simulink model "Commander_Stabilizer_Qdrone_wTrajTEMP"  (R2019a)
settings: Solver=ode2  StartTime=0.0  StopTime=inf  FixedStep=0.001  RelTol=1e-3  EnableMultiTasking=on
InitFcn:
  | set_param(gcs, 'ZoomFactor','FitSystem')
model workspace (MAT data in the model file):
  target_system = 1
undefined symbols (not defined in the file or in its folder): acc_calib, HIL
libraries: quarc_library x50, simulink x20, control_library x13, estimation_library x7
(part 1 of 3)
settings Model: SimulationMode=external  ExtModeTrigDuration=10000  Creator=dmadill  LastModifiedBy=user
settings SolverCC: PositivePriorityOrder=on
settings DataIOCC: LimitDataPoints=on  SaveFormat=Array  ReturnWorkspaceOutputs=off
settings OptimizationCC: LifeSpan=inf
settings DebuggingCC: SolverPrmCheckMsg=warning  SFUnexpectedBacktrackingDiag=warning  SFNoUnconditionalDefaultTransitionDiag=warning  SFExecutionAtInitializationDiag=none  ArithmeticOperatorsInVariantConditions=warning
settings HardwareCC: ProdBitPerLong=64  ProdLargestAtomicFloat=None  ProdHWDeviceType=Intel->x86-64
settings ModelReferenceCC: PropagateSignalLabelsOutOfModel=off
settings SFSimCC: SimUseLocalCustomCode=off
settings RTWCC: SystemTargetFile=quarc_linux_x64.tlc  TemplateMakefile=quarc_linux_x64_tmf  Description=QUARC Linux x64 Target  RTWUseLocalCustomCode=off
settings CodeAppCC: StateflowObjectComments=on
settings STFCustomTargetCC: TargetLibSuffix=.a  TargetPreCompLibLocation=C:\PROGRA~3\QUARC\lib\2019a\LINUX_~1\release  ConcurrentExecutionCompliant=on  SystemTargetFile=quarc_linux_x64.tlc
settings GRTTargetCC: TargetLibSuffix=.a  TargetPreCompLibLocation=C:\PROGRA~3\QUARC\lib\2019a\LINUX_~1\release  TargetLangStandard=C89/C90 (ANSI)  ParMdlRefBuildCompliant=off  CompOptLevelCompliant=off  CombineOutputUpdateFcns=off  MatFileLogging=off  CPPClassGenCompliant=off  GRTInterface=on  UseToolchainInfoCompliant=off  ExtMode=on  ExtModeMexFile=quarc_comm  ExtModeMexArgs='-w -d /tmp -uri %u -IP_address tcpip://192.168.1.157:18000', 'tcpip://192.168.1.25:17001?retries=10'
settings ConfigComp: CovMetricSettings=dw  CovHtmlReporting=on  CovSaveCumulativeToWorkspaceVar=on  CovSaveSingleToWorkspaceVar=on  CovExternalEMLEnable=off  CovSFcnEnable=off

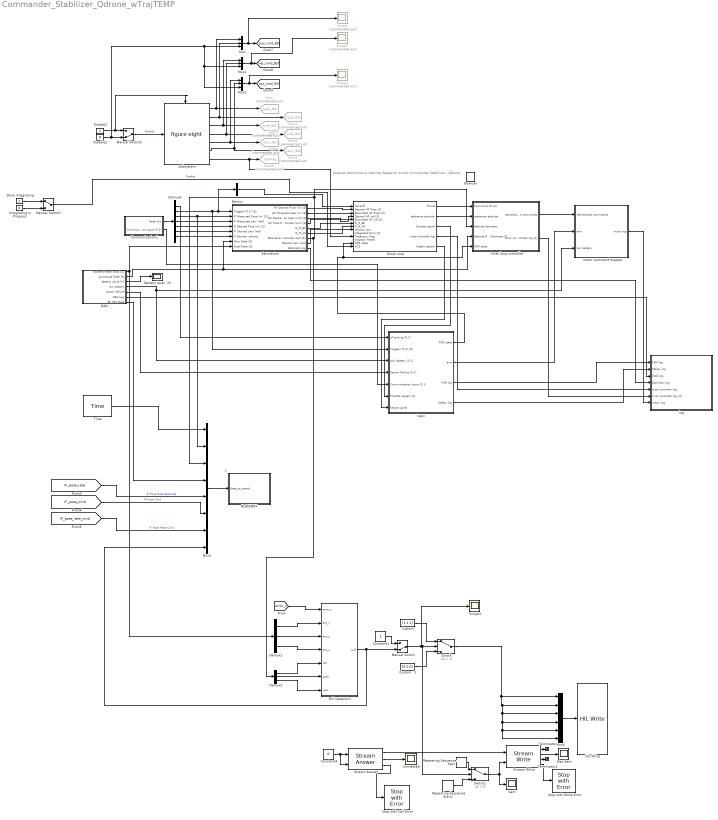
== system Commander_Stabilizer_Qdrone_wTrajTEMP ==
  note: Quanser Autonomous Vehicles Research Studio
      | Commander Stabilizer - QDrone
  note: 5
  "   Custom   " : Constant  Value=[1 1 1]
  "   Custom   1" : Constant  Value=[0 0 0]
  BLACKBOX : Subsystem
  Battery level  (V) : Scope
  Communication1 : Subsystem
  Connected : Scope
  Constant1 : Constant
  Constant4 : Constant  Value=0
  "DAQ " : Subsystem
  Demux : Demux  Outputs=3
  Demux1 : Demux  Outputs=3
  Demux2 : Demux  Outputs=3
  Demux5 : Demux  Outputs=[1 3 3 1 3 1 3]
  Disable2 : Constant  Value=0
  Done Integrating : Constant
  Enable2 : Constant
  "Estimation " : Subsystem
  Goto : Goto  Commented=on  GotoTag=xpos_8sh  TagVisibility=global
  Goto1 : Goto  Commented=on  GotoTag=ypos_8sh  TagVisibility=global
  Goto2 : Goto  Commented=on  GotoTag=xvel_8sh  TagVisibility=global
  Goto3 : Goto  Commented=on  GotoTag=yvel_8sh  TagVisibility=global
  Goto4 : Goto  Commented=on  GotoTag=xacc_8sh  TagVisibility=global
  Goto5 : Goto  Commented=on  GotoTag=yacc_8sh  TagVisibility=global
  Goto6 : Goto  Commented=on  GotoTag=trajFlag  TagVisibility=global
  HIL Write : quarc_library/Data Acquisition/Generic/Immediate I//O/HIL Write  object_name=HIL-1  analog_channels=[]  pwm_channels=[]  digital_channels=[5:7 9:23]  other_channels=[]  sample_time=-1  active=off  vector_input=on
      settings: SourceProductName=The database C:\Users\user\AppData\Roaming\MathWorks\MATLAB\R2017a\slblocks_master.db is locked, or a table in the database is locked. (database is locked)
  "Inner loop controller " : Subsystem
  Integrating in Progress : Constant  Value=0
  Manual Switch : ManualSwitch  CurrentSetting=0
  Manual Switch1 : ManualSwitch
  Manual Switch3 : ManualSwitch  CurrentSetting=0
  Mux : Mux  Inputs=3
  Mux1 : Mux  Inputs=3
  Mux2 : Mux  Inputs=3
  Mux3 : Mux  Inputs=[1 3 3 6 3 3 3 1]
  Mux4 : Mux  Inputs=6
  Outer loop : Subsystem
  Pull Detector1 : Subsystem
  Quanser : quarc_library/Logos/Quanser
  Repeating Sequence Stair : simulink/Sources/Repeating Sequence Stair  OutValues=[255 255 1 7 3 30 0 0 0 0 214].'  tsamp=-1  OutMin=[0]  OutMax=[]  OutDataTypeStr=fixdt(0,8,0)  OutputDataTypeScalingMode=Specify via dialog  OutDataType=fixdt(0,8,0)  ConRadixGroup=Best Precision: Vector-wise  OutScaling=[]
  Repeating Sequence Stair1 : simulink/Sources/Repeating Sequence Stair  OutValues=[255 255 1 7 3 30 255 3 0 0 212].'  tsamp=-1  OutMin=[0]  OutMax=[]  OutDataTypeStr=fixdt(0,8,0)  OutputDataTypeScalingMode=Specify via dialog  OutDataType=fixdt(0,8,0)  ConRadixGroup=Best Precision: Vector-wise  OutScaling=[]
  Scope : Scope  Commented=on
  Scope1 : Scope  Commented=on
  Scope2 : Scope  Commented=on
  Scope3 : Scope
  Sent : Scope
  Stop with Call Error : quarc_library/Sinks/Error Handling/Stop with Error  message_type=Interpret input as error code  message=Error occurred
      settings: SourceProductName=QUARC Targets
  Stop with Write Error : quarc_library/Sinks/Error Handling/Stop with Error  message_type=Interpret input as error code  message=Error occurred
      settings: SourceProductName=QUARC Targets
  Stream Answer : quarc_library/Communications/Intermediate/Stream Answer  uri_source=Specify via dialog (do not evaluate)  uri=serial://localhost:1?sndsize='16',baud='9600',word='8'  apply_uri_to_all_configs=on  send_buffer_size=128  receive_buffer_size=128  byte_order=little endian (Intel - LSB first)  sample_time=qc_get_step_size  active=off
      settings: AttributesFormatString="\"serial://localhost:1?sndsize='16',baud='9600',word='8'\""  SourceProductName=QUARC Targets
  Stream Write : quarc_library/Communications/Intermediate/Stream Write  optimization=Minimizing latency  send_dims=off
      settings: SourceProductName=QUARC Targets
  Subsystem : control_library/figure eight  TrajTime=8
  Switch : Switch  Criteria=u2 > Threshold
  Switch1 : Switch  Criteria=u2 > Threshold
  Terminator : Terminator
  Terminator1 : Terminator
  Time : quarc_library/Sources/Time/Time  time_source=Wall clock  sample_time=qc_get_step_size
  Was Sent : Scope
  "log " : Subsystem
  logic : Subsystem
  motor command mapper : Subsystem
  tag scope: acc_cmd_8sh=global, pos_cmd_8sh=global, vel_cmd_8sh=global
  wires:
  Demux5/3 -> "Estimation "/2(IF Measured Pose (m) [3]), Mux3/2
  Communication1/1(Data Out) -> Demux5/1
  Demux5/2 -> logic/2(Triggers (0,1) [3]), Demux/1, "Estimation "/1(Triggers (0,1) [3])
  "DAQ "/1(accelerometer Data [3]) -> "Estimation "/8(Accel Data [3]), Demux1/1
  Demux5/5 -> "Estimation "/4(IF Desired Pose (m) [3])
  Demux5/7 -> "Estimation "/6(IF Desired velocity)
  Demux5/4 -> "Estimation "/3(IF Measured yaw (rad))
  Demux5/6 -> "Estimation "/5(IF Desired yaw (rad))
  "DAQ "/2("gyroscope Data [3] ") -> "Estimation "/7(Gyro Data [3]), "Inner loop controller "/4(Attitude Rate Estimate [3])
  "Estimation "/1(HF Desired Pose (m) [3]) -> Outer loop/2(Desired HF Pose [3])
  "Estimation "/2(HF Pose Estimate (m) [3]) -> Outer loop/3(Estimated HF Pose [3])
  "Estimation "/3(HF Desired Pose rate (m/s) [3]) -> Outer loop/4(Desired HF vel [3])
  "Estimation "/4(HF Pose Rate Estimate (m/s) [3]) -> Outer loop/5(Estimated HF vel [3])
  "Estimation "/6(IF_R_HF) -> Outer loop/7(IF_R_HF)
  Demux5/1 -> logic/1(isTracking (0,1))
  logic/1("FSM state ") -> Outer loop/12("FSM state "), "Inner loop controller "/5(FSM state)
  "DAQ "/5(sensor failure) -> logic/4(Sensor Failure (0,1))
  "DAQ "/4(low battery) -> logic/3(Low Battery (0,1)), motor command mapper/3(low battery)
  Outer loop/1(Thrust) -> "Inner loop controller "/1(Command thrust)
  Communication1/2(Communication Issue (0,1)) -> logic/5(Communication Issue (0,1))
  "Inner loop controller "/1(Generalized commands) -> motor command mapper/1(Generalized commands)
  logic/2(arm) -> motor command mapper/2(arm)
  Outer loop/2(reference attitude) -> "Inner loop controller "/2(reference attitude)
  "Estimation "/7(Attitude Estimate (rad) [3]) -> Demux2/1, Mux3/3, "Inner loop controller "/3(Attitude Estimate)
  "DAQ "/6(DAQ Log) -> "log "/3(DAQ Log)
  "Estimation "/9(Estimator log) -> "log "/4(Estimator log)
  motor command mapper/1(motor log) -> "log "/7(motor log)
  Outer loop/4("outer controler log ") -> "log "/5("outer controler log ")
  "Inner loop controller "/2(inner controller log [4]) -> "log "/6(inner controller log [4])
  logic/3("FSM log ") -> "log "/1(FSM log)
  logic/4(Safety log) -> "log "/2(Safety log)
  "DAQ "/3(Battery Level (V)) -> Battery level  (V)/1
  Outer loop/5(height signals) -> logic/7(height signal)
  "Estimation "/5(IF_R_BF) -> Outer loop/6(IF_R_BF)
  "Estimation "/8(Desired Yaw (rad)) -> Outer loop/8(desired yaw)
  Outer loop/3(throttle signal) -> logic/6(Throttle signals [3])
  Manual Switch3/1 -> Subsystem/1  "Enable"
  Subsystem/5 -> Mux2/1, Goto4/1
  Mux/1 -> Scope/1, [pos_cmd_8sh]
  Mux1/1 -> Scope1/1, [vel_cmd_8sh]
  Subsystem/7 -> Outer loop/10(Trajectory Flag), Goto6/1
  Subsystem/6 -> Goto5/1, Mux2/2
  Subsystem/3 -> Mux1/1, Goto2/1
  Mux2/1 -> Scope2/1, [acc_cmd_8sh]
  Subsystem/4 -> Mux1/2, Goto3/1
  Disable2/1 -> Manual Switch3/2, Mux2/3, Mux1/3, Mux/3
  Subsystem/1 -> Mux/1, Goto/1
  Subsystem/2 -> Mux/2, Goto1/1
  Enable2/1 -> Manual Switch3/1, Subsystem/Enable
  Mux3/1 -> BLACKBOX/1("data_to_rocard ")
  Time/1 -> Mux3/1
  "DAQ "/7(BF IMU Data) -> Mux3/4
  [IF_pose_rate] -> Mux3/5  "IF Pose Rate Estimate"
  [IF_pose_cmd] -> Mux3/6  "IF Pose Cmd"
  [IF_pose_rate_cmd] -> Mux3/7  "IF Pose Rate Cmd"
  Demux/2 -> Outer loop/1(Takeoff)
  Done Integrating/1 -> Manual Switch1/1
  Integrating in Progress/1 -> Manual Switch1/2
  Manual Switch1/1 -> Outer loop/13(In13)  "Enable"
  Stream Write/1 -> Terminator/1
  Stream Answer/1 -> Stream Write/1
  Pull Detector1/1(pull) -> Mux3/8, Manual Switch/2
  Stream Write/2 -> Was Sent/1
  Repeating Sequence Stair1/1 -> Switch1/3
  Switch1/1 -> Stream Write/2, Sent/1
  Stream Answer/2 -> Connected/1
  Stream Write/4 -> Stop with Write Error/1
  Repeating Sequence Stair/1 -> Switch1/1
  Constant4/1 -> Stream Answer/1, Stream Answer/2
  Stream Answer/3 -> Stop with Call Error/1
  Constant1/1 -> Manual Switch/1
  Manual Switch/1 -> Switch1/2, Switch/2, Scope3/1
  "   Custom   1"/1 -> Switch/3
  Mux4/1 -> HIL Write/1
  "   Custom   "/1 -> Switch/1
  Switch/1 -> Mux4/6, Mux4/5, Mux4/4, Mux4/3, Mux4/2, Mux4/1
  Stream Write/3 -> Terminator1/1
  [error_z] -> Pull Detector1/1(error_z)
  Demux1/1 -> Pull Detector1/2(acc_x)
  Demux1/2 -> Pull Detector1/3(acc_y)
  Demux1/3 -> Pull Detector1/4(acc_z)
  Demux2/1 -> Pull Detector1/5(roll)
  Demux2/2 -> Pull Detector1/6(pitch)
  Demux2/3 -> Pull Detector1/7(yaw)

== system Commander_Stabilizer_Qdrone_wTrajTEMP/BLACKBOX ==
  "data_to_rocard " : Inport
  To Host File : quarc_library/Sinks/To Host/To Host File  file_name=saved_data/%m/record_data_%{date}_%{time}.mat  variable_name=optitack_imu_data  decimation=1  sample_time=-1  file_format=MAT-file v.5  options=No header or footer  append=off  final_file_name=saved_data/Commander_Stabilizer_Qdrone_wTrajTEMP/record_data_30-Mar-2021_18-24-55.mat  bitrate=2000000
  wires:
  "data_to_rocard "/1 -> To Host File/1

== system Commander_Stabilizer_Qdrone_wTrajTEMP/Communication1 ==
  note: Argument (- IP_address ) is set at the MEX-file arguments found at Model Configuration Properties > Code Generation > Interface
      |
      | Format:
      | tcpip://192.168.2.H:18000
      | where H is the last digits of your ground station's IP address (use ipconfig in a command prompt to find it out).
  Constant : Constant
  Detect Communication Loss : Subsystem
  Memory : Memory  InheritSampleTime=on  LinearizeMemory=on  LinearizeAsDelay=on
  Model Argument : quarc_library/Sources/Signals/Model Argument  argument_name=IP_address  has_value=on  data_type_mode=Specify via dialog  data_type=char  max_length=80  variable_size=off
      settings: AttributesFormatString=(-%<argument_name>)  SourceProductName=QUARC Targets
  Select Timestamp received and send back immediately (for calculating loopback time) : Selector  InputPortWidth=16  IndexOptions=Index vector (dialog)  Indices=[16]  OutputSizes=1
  Select the rest of the data : Selector  InputPortWidth=16  IndexOptions=Index vector (dialog)  Indices=[1:15]  OutputSizes=1
  Stream Client : quarc_library/Communications/Basic/Stream Client  uri_source=External input port  uri=tcpip://192.168.2.3:18669  apply_uri_to_all_configs=on  send_buffer_size=128  receive_buffer_size=128  byte_order=little endian (Intel - LSB first)  optimization=Minimum latency  send_options=Send most recent data  receive_options=Receive most recent data  default_value=zeros(1,16)  sample_time=qc_get_step_size  active=off  implementation=Use blocking I/O in a separate thread  send_fifo_size=128  receive_fifo_size=128  send_priority=0  receive_priority=0  send_dimensions=off  receive_dimensions=off  max_dimensions=-1  data_type=Inherited via back propagation  type_expr=BusObject
  String Display : quarc_library/Strings/String Display  alignment=center  display_mode=Single line  sample_time=-1
      settings: SourceProductName=QUARC Targets
  Terminator1 : Terminator
  Terminator2 : Terminator
  Data Out : Outport
  Communication Issue (0,1) : Outport  Port=2
  wires:
  Stream Client/5 -> Terminator2/1
  Model Argument/1 -> Stream Client/3, String Display/1
  Constant/1 -> Stream Client/2
  Stream Client/3 -> Terminator1/1
  Stream Client/4 -> Detect Communication Loss/3(Data Out), Select Timestamp received and send back immediately (for calculating loopback time)/1, Select the rest of the data/1
  Memory/1 -> Stream Client/1
  Stream Client/1 -> Detect Communication Loss/1(State)
  Stream Client/2 -> Detect Communication Loss/2(Error)
  Detect Communication Loss/1(Communication Issue) -> Communication Issue (0,1)/1
  Select the rest of the data/1 -> Data Out/1
  Select Timestamp received and send back immediately (for calculating loopback time)/1 -> Memory/1

== system Commander_Stabilizer_Qdrone_wTrajTEMP/DAQ  ==
  note: Read the sensors and battery voltage
  note: Gyro and Accel data rate at 1000Hz
  Accel (m/s/s) [3] : Selector  InputPortWidth=6  IndexOptions=Index vector (dialog)  Indices=[4:6]  OutputSizes=1
  "Battery Level, Accelrometer and Gyroscope" : quarc_library/Data Acquisition/Generic/Immediate I//O/HIL Read  Priority=1  object_name=HIL-1  analog_channels=[4]  encoder_channels=[]  digital_channels=[]  other_channels=[3000:3002 4000:4002]  sample_time=qc_get_step_size  active=on  vector_output=on  data_type_mode=Inherit via back propagation  encoder_data_type=double  digital_data_type=boolean
      settings: SourceProductName=The database C:\Users\user\AppData\Roaming\MathWorks\MATLAB\R2017a\slblocks_master.db is locked, or a table in the database is locked. (database is locked)
  Check Battery level : Subsystem
  Conversion : Gain  Gain=11.2
  Gyro (rad/s) [3] : Selector  InputPortWidth=6  IndexOptions=Index vector (dialog)  Indices=[1:3]  OutputSizes=1
  HIL Initialize : quarc_library/Data Acquisition/Generic/Configuration/HIL Initialize  object_name=HIL-1  board_type=qdrone  board_number=0  board_options=gyro_fs=2000;gyro_rate=1000;gyro_os=4;accel_fs=16;accel_rate=400;accel_os=4;baro_os=4096  exclusive=off  active=on  hardware_clocks=[]  clock_modes=[]  initial_clock_frequencies=[]  set_clock_params_at_start=off  set_clock_params_at_switch_in=off  set_clock_frequencies_at_start=off  set_clock_frequencies_at_switch_in=off  analog_input_channels=[0:4]  analog_input_configurations=[]  analog_input_maximums=[3.3]  analog_input_minimums=[0]  set_analog_input_params_at_start=off  set_analog_input_params_at_switch_in=off  analog_output_channels=[]  analog_output_maximums=[]  analog_output_minimums=[]  initial_analog_outputs=[]  final_analog_outputs=[]  watchdog_analog_outputs=[]  set_analog_output_params_at_start=off  set_analog_output_params_at_switch_in=off  set_analog_outputs_at_start=off  set_analog_outputs_at_switch_in=off  set_analog_outputs_at_terminate=off  set_analog_outputs_at_switch_out=off  set_analog_outputs_on_watchdog=off  digital_input_channels=[]  digital_output_channels=[5:7 9:23]  digital_output_configuration=[]  initial_digital_outputs=[0]  final_digital_outputs=[0]  watchdog_digital_outputs=[]  set_digital_output_params_at_start=off  set_digital_output_params_at_switch_in=off  set_digital_outputs_at_start=on  set_digital_outputs_at_switch_in=off  set_digital_outputs_at_terminate=on  set_digital_outputs_at_switch_out=off  set_digital_outputs_on_watchdog=off  encoder_channels=[0:2]  quadrature=[4]  encoder_filter_frequency=50e6/1  initial_encoder_counts=[0]  set_encoder_params_at_start=on  set_encoder_params_at_switch_in=off  set_encoder_counts_at_start=on  set_encoder_counts_at_switch_in=off  pwm_channels=[0:3]  pwm_modes=[4]  pwm_frequency=2000  pwm_configuration=[0]  pwm_alignment=[0]  pwm_polarity=[1]  pwm_leading_deadband=[]  pwm_trailing_deadband=[]  initial_pwm_outputs=[0]  final_pwm_outputs=[0]  watchdog_pwm_outputs=[0]  set_pwm_params_at_start=on  set_pwm_params_at_switch_in=off  set_pwm_outputs_at_start=on  set_pwm_outputs_at_switch_in=off  set_pwm_outputs_at_terminate=on  set_pwm_outputs_at_switch_out=off  set_pwm_outputs_on_watchdog=off  other_output_channels=[]  initial_other_outputs=[]  final_other_outputs=[]  watchdog_other_outputs=[]  set_other_outputs_at_start=off  set_other_outputs_at_switch_in=off  set_other_outputs_at_terminate=off  set_other_outputs_at_switch_out=off  set_other_outputs_on_watchdog=off
      settings: SourceProductName=The database C:\Users\user\AppData\Roaming\MathWorks\MATLAB\R2017a\slblocks_master.db is locked, or a table in the database is locked. (database is locked)
  Mux : Mux  Inputs=5
  Sensor Failure Monitoring : Subsystem
  accelerometer Data [3] : Outport
  "gyroscope Data [3] " : Outport  Port=2
  Battery Level (V) : Outport  Port=3
  low battery : Outport  Port=4
  sensor failure : Outport  Port=5
  DAQ Log : Outport  Port=6
  BF IMU Data : Outport  Port=7
  wires:
  Mux/1 -> DAQ Log/1
  Sensor Failure Monitoring/1(Sensor Failure) -> sensor failure/1, Mux/1
  Accel (m/s/s) [3]/1 -> accelerometer Data [3]/1, Sensor Failure Monitoring/2(Accel Data [3]1), Mux/5
  "Battery Level, Accelrometer and Gyroscope"/2 -> BF IMU Data/1, Accel (m/s/s) [3]/1, Gyro (rad/s) [3]/1
  Check Battery level/1(Low Battery) -> low battery/1, Mux/3
  "Battery Level, Accelrometer and Gyroscope"/1 -> Conversion/1
  Conversion/1 -> Mux/2, Battery Level (V)/1, Check Battery level/1(Battery level)
  Gyro (rad/s) [3]/1 -> "gyroscope Data [3] "/1, Sensor Failure Monitoring/1(Gyro Data [3]), Mux/4

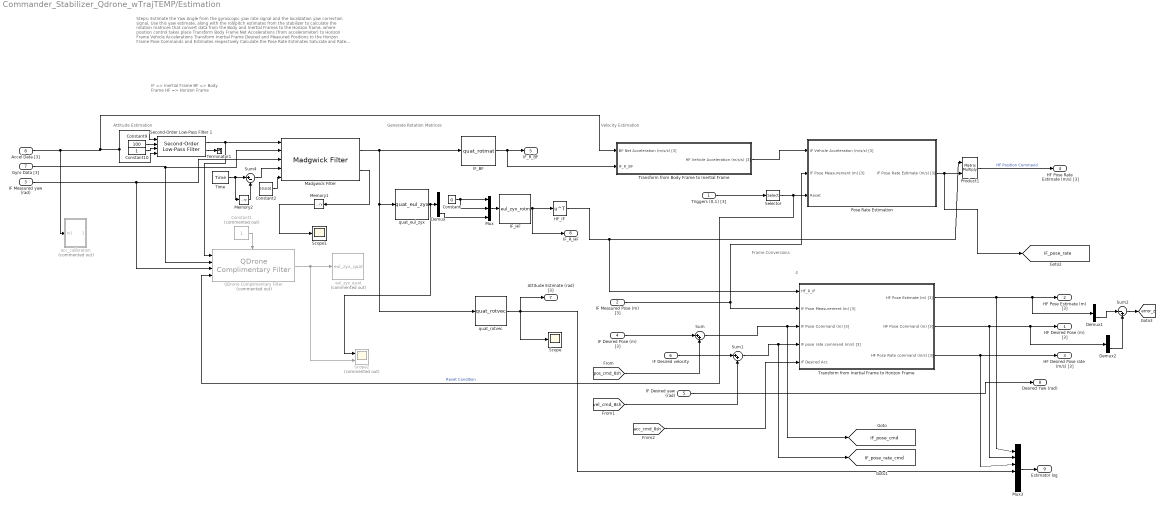
== system Commander_Stabilizer_Qdrone_wTrajTEMP/Estimation  ==
  note: IF => Inertial Frame
      | BF => Body Frame
      | HF => Horizon Frame
  note: 4
  note: Steps:
      |
      | Estimate the Yaw Angle from the gyroscopic yaw rate signal and the localization yaw correction signal.
      | Use this yaw estimate, along with the roll/pitch estimates from the stabilizer to calculate the rotation matrices that convert data from the Body and Inertial Frames to the Horizon frame, where position control takes place
      | Transform Body Frame Net Accelerations (from accelerometer) to Horizon Frame Vehicle Accelerations
      | Transform Inertial Frame Desired and Measured Positions to the Horizon Frame Pose Commands and Estimates respectively
      | Calculate the Pose Rate Estimates
      | Saturate and Rate Limit the IF Desired Pose based on workspace limitations
  note: Attitude Estimation
  note: Generate Rotation Matrices
  note: Velocity Estimation
  note: Frame Conversions
  Triggers (0,1) [3] : Inport
  IF Measured Pose (m) [3] : Inport  Port=2
  IF Measured yaw (rad) : Inport  Port=3
  IF Desired Pose (m) [3] : Inport  Port=4
  IF Desired yaw (rad) : Inport  Port=5
  IF Desired velocity : Inport  Port=6
  Gyro Data [3] : Inport  Port=7
  Accel Data [3] : Inport  Port=8
  Constant : Constant  Value=0
  Constant1 : Constant  Commented=on
  Constant10 : Constant
  Constant2 : Constant  Value=[0;0;0]
  Constant9 : Constant  Value=100
  Demux : Demux  Outputs=3
  Demux1 : Demux  Outputs=3
  Demux2 : Demux  Outputs=3
  HF_IF : Math  Operator=transpose  SaturateOnIntegerOverflow=on
  IF_BF : estimation_library/quat_rotmat
  IF_HF : estimation_library/eul_zyx_rotm
  Madgwick Filter : estimation_library/Madgwick Filter  beta=0.0453*0.1  zeta=0  acc_tol=1.1*9.78909*1e3
  Memory1 : Memory  InitialCondition=[0, 0, 0]  InheritSampleTime=on
  Memory2 : Memory  InheritSampleTime=on
  Mux : Mux  Inputs=3
  Mux3 : Mux  Inputs=6
  Pose Rate Estimation : Subsystem
  Product1 : Product  Multiplication=Matrix(*)
  QDrone Complimentary Filter : estimation_library/QDrone Complimentary Filter  Commented=on  SystemSampleTime=-1
  Scope : Scope
  Scope1 : Scope
  Scope2 : Scope  Commented=on  NumInputPorts=2
  Second-Order Low-Pass Filter 1 : quarc_library/Continuous/Second-Order Low-Pass Filter  params_source=External (input ports)  input_width=50  input_zeta=1  input_init=0
      settings: SourceProductName=The database C:\Users\user\AppData\Roaming\MathWorks\MATLAB\R2017a\slblocks_master.db is locked, or a table in the database is locked. (database is locked)
  Selector : Selector  InputPortWidth=3  IndexOptions=Index vector (dialog)  Indices=[2]  OutputSizes=1
  Sum : Sum  Inputs=|++
  Sum1 : Sum  Inputs=|++
  Sum2 : Sum  Inputs=|-+
  Sum4 : Sum  Inputs=|+-
  Terminator1 : Terminator
  Time : quarc_library/Sources/Time/Time  time_source=Wall clock  sample_time=qc_get_step_size
  Transform from Body Frame to Inertial Frame : Subsystem
  Transform from Inertial Frame to Horizon Frame : Subsystem
  acc_calibration : Subsystem  Commented=on
  eul_zyx_quat : estimation_library/eul_zyx_quat  Commented=on
  quat_eul_zyx : estimation_library/quat_eul_zyx
  quat_rotvec : estimation_library/quat_rotvec
  HF Desired Pose (m) [3] : Outport
  HF Pose Estimate (m) [3] : Outport  Port=2
  HF Desired Pose rate (m/s) [3] : Outport  Port=3
  HF Pose Rate Estimate (m/s) [3] : Outport  Port=4
  IF_R_BF : Outport  Port=5
  IF_R_HF : Outport  Port=6
  Attitude Estimate (rad) [3] : Outport  Port=7
  Desired Yaw (rad) : Outport  Port=8
  Estimator log : Outport  Port=9
  tag scope: IF_pose_cmd=global, IF_pose_rate=global, IF_pose_rate_cmd=global, error_z=global
  wires:
  IF Measured Pose (m) [3]/1 -> Transform from Inertial Frame to Horizon Frame/2(IF Pose Measurement (m) [3]), Pose Rate Estimation/2(IF Pose Measurement (m) [3])
  Triggers (0,1) [3]/1 -> Selector/1
  Transform from Inertial Frame to Horizon Frame/2(HF Pose Command (m) [3]) -> Mux3/2, Demux2/1, HF Desired Pose (m) [3]/1
  Transform from Body Frame to Inertial Frame/1(HF Vehicle Acceleration (m/s/s) [3]) -> Pose Rate Estimation/1(IF Vehicle Acceleration (m/s/s) [3])
  Selector/1 -> QDrone Complimentary Filter/4, Pose Rate Estimation/3(Reset)  "Reset Condition"
  IF Desired Pose (m) [3]/1 -> Sum/1
  IF Desired velocity/1 -> Sum1/1
  Transform from Inertial Frame to Horizon Frame/3(HF Pose Rate command (m/s) [3]) -> HF Desired Pose rate (m/s) [3]/1, Mux3/3
  Memory2/1 -> Sum4/2
  Time/1 -> Memory2/1, Sum4/1
  Sum4/1 -> Madgwick Filter/4
  Madgwick Filter/2 -> Memory1/1
  Gyro Data [3]/1 -> Madgwick Filter/2, QDrone Complimentary Filter/2
  quat_eul_zyx/1 -> Scope2/1, Demux/1
  Constant/1 -> Mux/2, Mux/1
  Mux/1 -> IF_HF/1
  IF_HF/1 -> IF_R_HF/1, HF_IF/1
  HF_IF/1 -> Product1/1, Transform from Inertial Frame to Horizon Frame/1(HF_R_IF)
  Constant10/1 -> Second-Order Low-Pass Filter 1/3
  Constant9/1 -> Second-Order Low-Pass Filter 1/2
  Second-Order Low-Pass Filter 1/1 -> Madgwick Filter/1, QDrone Complimentary Filter/1
  Second-Order Low-Pass Filter 1/2 -> Terminator1/1
  Mux3/1 -> Estimator log/1
  Transform from Inertial Frame to Horizon Frame/1(HF Pose Estimate (m) [3]) -> Demux1/1, HF Pose Estimate (m) [3]/1, Mux3/1
  quat_rotvec/1 -> Attitude Estimate (rad) [3]/1, Scope/1, Mux3/4
  Memory1/1 -> Scope1/1
  IF Desired yaw (rad)/1 -> Desired Yaw (rad)/1
  IF Measured yaw (rad)/1 -> Madgwick Filter/3, QDrone Complimentary Filter/3
  Constant1/1 -> QDrone Complimentary Filter/Enable
  QDrone Complimentary Filter/1 -> Scope2/2, eul_zyx_quat/1
  Product1/1 -> HF Pose Rate Estimate (m/s) [3]/1  "HF Position Command"
  IF_BF/1 -> Transform from Body Frame to Inertial Frame/2(IF_R_BF), IF_R_BF/1
  Demux/3 -> Mux/3
  Pose Rate Estimation/1(IF Pose Rate Estimate (m/s) [3]) -> [IF_pose_rate], Product1/2
  Sum/1 -> [IF_pose_cmd], Transform from Inertial Frame to Horizon Frame/3(IF Pose Command (m) [3])
  [pos_cmd_8sh] -> Sum/2
  Sum1/1 -> [IF_pose_rate_cmd], Transform from Inertial Frame to Horizon Frame/4(IF pose rate command (m/s) [3])
  [vel_cmd_8sh] -> Sum1/2
  [acc_cmd_8sh] -> Transform from Inertial Frame to Horizon Frame/5(IF Desired Acc)
  Constant2/1 -> Madgwick Filter/5
  Accel Data [3]/1 -> acc_calibration/1(In1), Second-Order Low-Pass Filter 1/1, Second-Order Low-Pass Filter 1/4, Transform from Body Frame to Inertial Frame/1(BF Net Acceleration (m/s/s) [3])
  Sum2/1 -> [error_z]
  Demux2/3 -> Sum2/2
  Demux1/3 -> Sum2/1
  Madgwick Filter/1 -> quat_rotvec/1, quat_eul_zyx/1, IF_BF/1

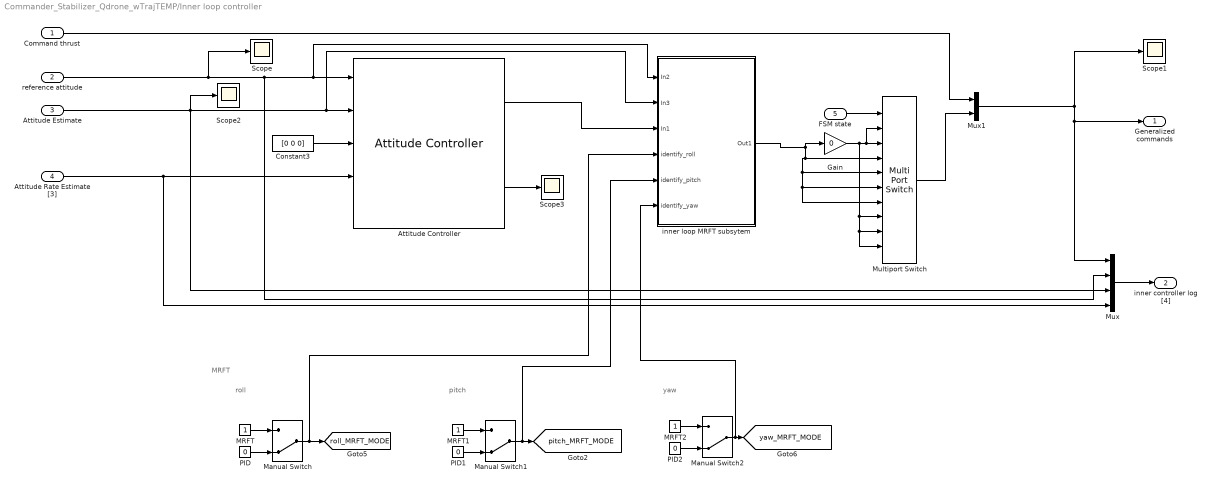
== system Commander_Stabilizer_Qdrone_wTrajTEMP/Inner loop controller  ==
  note: MRFT
  note: pitch
  note: roll
  note: yaw
  Command thrust : Inport
  reference attitude : Inport  Port=2
  Attitude Estimate : Inport  Port=3
  Attitude Rate Estimate [3] : Inport  Port=4
  FSM state : Inport  Port=5
  Attitude Controller : control_library/Attitude Controller  P_x=1.3852  I_x=0  D_x=0.1564  P_y=1.3542  I_y=0  D_y=0.1529  P_z=0.6  I_z=0  D_z=0.12  velRef=off  LowPassPID=off  T_lowpass=0
  Constant3 : Constant  Value=[0 0 0]
  Gain : Gain  Gain=0
  MRFT : Constant
  MRFT1 : Constant
  MRFT2 : Constant
  Manual Switch : ManualSwitch  CurrentSetting=0
  Manual Switch1 : ManualSwitch  CurrentSetting=0
  Manual Switch2 : ManualSwitch  CurrentSetting=0
  Multiport Switch : MultiPortSwitch  Inputs=9
  Mux : Mux
  Mux1 : Mux  Inputs=2
  PID : Constant  Value=0
  PID1 : Constant  Value=0
  PID2 : Constant  Value=0
  Scope{,1..3} (4 alike) : Scope
  inner loop MRFT subsytem : Subsystem
  Generalized commands : Outport
  inner controller log [4] : Outport  Port=2
  tag scope: pitch_MRFT_MODE=global, roll_MRFT_MODE=global, yaw_MRFT_MODE=global
  wires:
  Constant3/1 -> Attitude Controller/3
  reference attitude/1 -> Scope/1, Mux/2, inner loop MRFT subsytem/1(In2), Attitude Controller/1
  Command thrust/1 -> Mux1/1
  Mux/1 -> inner controller log [4]/1
  Attitude Rate Estimate [3]/1 -> Attitude Controller/4, Mux/4
  Attitude Controller/2 -> Scope3/1
  Attitude Estimate/1 -> inner loop MRFT subsytem/2(In3), Attitude Controller/2, Mux/3, Scope2/1
  Mux1/1 -> Mux/1, Generalized commands/1, Scope1/1
  FSM state/1 -> Multiport Switch/1
  Gain/1 -> Multiport Switch/10, Multiport Switch/9, Multiport Switch/8, Multiport Switch/3, Multiport Switch/2
  Multiport Switch/1 -> Mux1/2
  MRFT1/1 -> Manual Switch1/1
  Manual Switch/1 -> inner loop MRFT subsytem/4(identify_roll), [roll_MRFT_MODE]
  Manual Switch2/1 -> inner loop MRFT subsytem/6(identify_yaw), [yaw_MRFT_MODE]
  MRFT2/1 -> Manual Switch2/1
  PID/1 -> Manual Switch/2
  MRFT/1 -> Manual Switch/1
  PID1/1 -> Manual Switch1/2
  PID2/1 -> Manual Switch2/2
  Manual Switch1/1 -> inner loop MRFT subsytem/5("identify_pitch "), [pitch_MRFT_MODE]
  Attitude Controller/1 -> inner loop MRFT subsytem/3(In1)
  inner loop MRFT subsytem/1(Out1) -> Multiport Switch/7, Multiport Switch/6, Multiport Switch/5, Multiport Switch/4, Gain/1

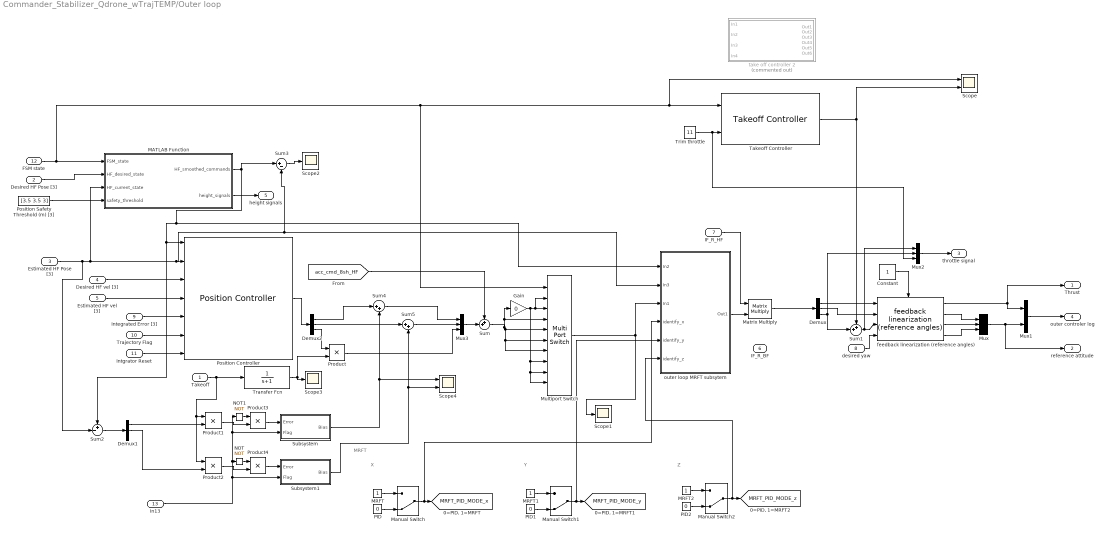
== system Commander_Stabilizer_Qdrone_wTrajTEMP/Outer loop ==
  note: X
  note: MRFT
  note: Y
  note: Z
  Takeoff : Inport
  Desired HF Pose [3] : Inport  Port=2
  Estimated HF Pose [3] : Inport  Port=3
  Desired HF vel [3] : Inport  Port=4
  Estimated HF vel [3] : Inport  Port=5
  IF_R_BF : Inport  Port=6
  IF_R_HF : Inport  Port=7
  desired yaw : Inport  Port=8
  Integrated Error [3] : Inport  Port=9
  Trajectory Flag : Inport  Port=10
  Intgrator Reset : Inport  Port=11
  "FSM state " : Inport  Port=12
  In13 : Inport  Port=13
  Constant : Constant
  Demux : Demux  Outputs=3
  Demux1 : Demux  Outputs=3
  Demux2 : Demux  Outputs=3
  Gain : Gain  Gain=0
  MATLAB Function : MATLAB Function  TreatAsAtomicUnit=on
  MRFT : Constant
  MRFT1 : Constant
  MRFT2 : Constant
  Manual Switch : ManualSwitch  CurrentSetting=0
  Manual Switch1 : ManualSwitch  CurrentSetting=0
  Manual Switch2 : ManualSwitch  CurrentSetting=0
  Matrix Multiply : Product  Multiplication=Matrix(*)
  Multiport Switch : MultiPortSwitch  Inputs=9
  Mux : Mux  Inputs=3
  Mux1 : Mux  Inputs=2
  Mux2 : Mux  Inputs=3
  Mux3 : Mux  Inputs=3
  NOT : Logic  Operator=NOT  IconShape=distinctive  AllPortsSameDT=off  OutDataTypeStr=boolean
  NOT1 : Logic  Operator=NOT  IconShape=distinctive  AllPortsSameDT=off  OutDataTypeStr=boolean
  PID : Constant  Value=0
  PID1 : Constant  Value=0
  PID2 : Constant  Value=0
  Position Controller : control_library/Position Controller  P_x=34.159  I_x=0  D_x=9.3766  P_x_traj=40.97  I_x_traj=86.7  D_x_traj=8.48  P_y=34.775  I_y=0  D_y=9.54  P_y_traj=40.97  I_y_traj=86.7  D_y_traj=8.48  P_z=166.7  I_z=0  D_z=25.9  P_z_traj=185.7  I_z_traj=0  D_z_traj=28.88  trajectoryGains=off  velRef=off  externalIntError=off  LowPassPID=off  T_lowpass=0
  Position Safety Threshold (m) [3] : Constant  Value=[3.5 3.5 3]
  Product{,1..4} (5 alike) : Product
  Scope : Scope  NumInputPorts=2
  Scope1 : Scope
  Scope2 : Scope
  Scope3 : Scope
  Scope4 : Scope  NumInputPorts=2
  Subsystem : Subsystem
  Subsystem1 : Subsystem
  Sum : Sum  Inputs=++|
  Sum1 : Sum  Inputs=++|
  Sum2 : Sum  Inputs=+-|
  Sum3 : Sum  Inputs=|+-
  Sum4 : Sum  Inputs=|++
  Sum5 : Sum  Inputs=|++
  Takeoff Controller : control_library/Takeoff Controller  SystemSampleTime=-1
      link override Saturation1: UpperLimit=[0 0]  LowerLimit=[0 0]
  Transfer Fcn : TransferFcn  Denominator=[1 1]
  Trim throttle : Constant  Value=11
  feedback linearization (reference angles) : control_library/feedback linearization (reference angles)  SystemSampleTime=-1
  outer loop MRFT subsytem : Subsystem
  take off controller 2 : Subsystem  Commented=on
  Thrust : Outport
  reference attitude : Outport  Port=2
  throttle signal : Outport  Port=3
  "outer controler log " : Outport  Port=4
  height signals : Outport  Port=5
  tag scope: MRFT_PID_MODE_x=global, MRFT_PID_MODE_y=global, MRFT_PID_MODE_z=global
  wires:
  Trajectory Flag/1 -> Position Controller/6
  Intgrator Reset/1 -> Position Controller/7
  Estimated HF vel [3]/1 -> Position Controller/4
  Desired HF vel [3]/1 -> Position Controller/3
  Integrated Error [3]/1 -> Position Controller/5
  Mux1/1 -> "outer controler log "/1
  "FSM state "/1 -> Multiport Switch/1, Scope/1, Takeoff Controller/1, MATLAB Function/1(FSM_state)
  MATLAB Function/1(HF_smoothed_commands) -> outer loop MRFT subsytem/1(In2), Sum2/1, Position Controller/1, Sum3/1
  Position Safety Threshold (m) [3]/1 -> MATLAB Function/4(safety_threshold)
  MATLAB Function/2(height_signals) -> height signals/1
  Trim throttle/1 -> Takeoff Controller/2, Mux2/3
  Mux2/1 -> throttle signal/1
  Sum1/1 -> feedback linearization (reference angles)/3, Mux2/1
  Takeoff Controller/1 -> Sum1/1, Scope/2
  Desired HF Pose [3]/1 -> MATLAB Function/2(HF_desired_state)
  feedback linearization (reference angles)/1 -> Mux1/1, Thrust/1
  Constant/1 -> feedback linearization (reference angles)/Enable
  feedback linearization (reference angles)/2 -> Mux/1
  feedback linearization (reference angles)/3 -> Mux/2
  Estimated HF Pose [3]/1 -> Sum2/2, MATLAB Function/3(HF_current_state), Sum3/2, outer loop MRFT subsytem/2(In3), Position Controller/2
  Mux/1 -> Mux1/2, reference attitude/1
  feedback linearization (reference angles)/4 -> Mux/3
  PID/1 -> Manual Switch/2
  MRFT/1 -> Manual Switch/1
  Manual Switch/1 -> outer loop MRFT subsytem/4(identify_x), [MRFT_PID_MODE_x]
  Manual Switch1/1 -> outer loop MRFT subsytem/5("identify_y "), [MRFT_PID_MODE_y]
  MRFT1/1 -> Manual Switch1/1
  PID1/1 -> Manual Switch1/2
  Manual Switch2/1 -> outer loop MRFT subsytem/6(identify_z), [MRFT_PID_MODE_z]
  MRFT2/1 -> Manual Switch2/1
  PID2/1 -> Manual Switch2/2
  outer loop MRFT subsytem/1(Out1) -> Matrix Multiply/2
  Matrix Multiply/1 -> Demux/1
  IF_R_HF/1 -> Matrix Multiply/1
  Demux/3 -> Sum1/2, Mux2/2
  desired yaw/1 -> feedback linearization (reference angles)/4
  Demux/1 -> feedback linearization (reference angles)/1
  Demux/2 -> feedback linearization (reference angles)/2
  Sum3/1 -> Scope2/1
  Mux3/1 -> Sum/2
  Gain/1 -> Multiport Switch/10, Multiport Switch/9, Multiport Switch/8, Multiport Switch/3, Multiport Switch/2
  Multiport Switch/1 -> outer loop MRFT subsytem/3(In1), Scope1/1
  Position Controller/1 -> Demux2/1
  Takeoff/1 -> Product1/1, Product2/1, Transfer Fcn/1
  Transfer Fcn/1 -> Scope3/1, Product/2
  Demux2/1 -> Sum4/1
  Demux2/2 -> Sum5/1
  Demux2/3 -> Product/1
  Product/1 -> Mux3/3
  Sum/1 -> Multiport Switch/4, Gain/1, Multiport Switch/6, Multiport Switch/7, Multiport Switch/5
  [acc_cmd_8sh_HF] -> Sum/1
  Demux1/2 -> Product2/2
  Sum2/1 -> Demux1/1
  Demux1/1 -> Product1/2
  Product1/1 -> Product3/2
  Product2/1 -> Product4/2
  Sum5/1 -> Mux3/2
  Sum4/1 -> Mux3/1
  Subsystem/1(Bias) -> Scope4/1, Sum4/2
  Subsystem1/1(Bias) -> Scope4/2, Sum5/2
  Product4/1 -> Subsystem1/1(Error)
  In13/1 -> Subsystem1/2(Flag), NOT/1, Subsystem/2(Flag), NOT1/1
  Product3/1 -> Subsystem/1(Error)
  NOT/1 -> Product4/1
  NOT1/1 -> Product3/1

== system Commander_Stabilizer_Qdrone_wTrajTEMP/Pull Detector1 ==
  error_z : Inport
  acc_x : Inport  Port=2
  acc_y : Inport  Port=3
  acc_z : Inport  Port=4
  roll : Inport  Port=5
  pitch : Inport  Port=6
  yaw : Inport  Port=7
  Constant : Constant  Value=50  OutDataTypeStr=single
  MATLAB Function : MATLAB Function  TreatAsAtomicUnit=on
  MATLAB Function1 : MATLAB Function  TreatAsAtomicUnit=on
  Scope4 : Scope  NumInputPorts=3
  pull : Outport  VectorParamsAs1DForOutWhenUnconnected=on
  wires:
  yaw/1 -> MATLAB Function/7(yaw)
  roll/1 -> MATLAB Function/5(roll)
  Constant/1 -> MATLAB Function1/2(threshold)
  acc_x/1 -> MATLAB Function/2(acc_x)
  acc_y/1 -> MATLAB Function/3(acc_y)
  MATLAB Function/1(detection_output) -> MATLAB Function1/1(u), Scope4/1
  acc_z/1 -> MATLAB Function/4(acc_z)
  pitch/1 -> MATLAB Function/6(pitch)
  error_z/1 -> Scope4/3, MATLAB Function/1(error_z)
  MATLAB Function1/1(y) -> Scope4/2, pull/1

== system Commander_Stabilizer_Qdrone_wTrajTEMP/log  ==
  FSM log : Inport
  Safety log : Inport  Port=2
  DAQ Log : Inport  Port=3
  Estimator log : Inport  Port=4
  "outer controler log " : Inport  Port=5
  inner controller log [4] : Inport  Port=6
  motor log : Inport  Port=7
  BLACKBOX : Subsystem
  BLACKBOX1 : Subsystem
  Inner loop MRFT : Subsystem
  "MRFT data concat " : Subsystem
  wires:
  FSM log/1 -> BLACKBOX/1(FSM Monitor Log)
  Estimator log/1 -> BLACKBOX/2(Estimator log)
  "MRFT data concat "/1(Out1) -> BLACKBOX/4(MRFT info)
  "outer controler log "/1 -> BLACKBOX/3(Controller Log)
  Safety log/1 -> BLACKBOX1/1(Safety Log)
  inner controller log [4]/1 -> BLACKBOX1/3(Controller log)
  motor log/1 -> BLACKBOX1/4(motor log)
  DAQ Log/1 -> BLACKBOX1/2(DAQ log)
  Inner loop MRFT/1(Out1) -> BLACKBOX1/5(MRFT log)

== system Commander_Stabilizer_Qdrone_wTrajTEMP/logic ==
  note: 1
  isTracking (0,1) : Inport
  Triggers (0,1) [3] : Inport  Port=2
  Low Battery (0,1) : Inport  Port=3
  Sensor Failure (0,1) : Inport  Port=4
  Communication Issue (0,1) : Inport  Port=5
  Throttle signals [3] : Inport  Port=6
  height signal : Inport  Port=7
  Constant : Constant  Value=0
  Display : Display
  FLIGHT SAFETY : Subsystem
  FSM MONITOR : Subsystem
  "FSM state " : Outport
  arm : Outport  Port=2
  "FSM log " : Outport  Port=3
  Safety log : Outport  Port=4
  wires:
  FLIGHT SAFETY/2(Emergency Land) -> FSM MONITOR/1(Land due to Health Issues (0,1))
  isTracking (0,1)/1 -> FSM MONITOR/5(isTracking (0,1))
  Low Battery (0,1)/1 -> FSM MONITOR/2(Low Battery (0,1))
  Communication Issue (0,1)/1 -> FSM MONITOR/4(Communication Issue (w/ MS))
  Sensor Failure (0,1)/1 -> FSM MONITOR/3(Sensor Failure (0,1))
  Triggers (0,1) [3]/1 -> FSM MONITOR/6(Triggers (0,1) [3])
  FSM MONITOR/3(Arm (0,1)) -> FLIGHT SAFETY/1(Arm), arm/1
  FSM MONITOR/2(Stop Model (0,1)) -> FLIGHT SAFETY/2(Stop Model)
  Throttle signals [3]/1 -> FSM MONITOR/7(Throttle Signals (N) [3])
  FSM MONITOR/4(FSM State (0-9)) -> "FSM state "/1
  FSM MONITOR/1(FSM Monitor Log) -> "FSM log "/1
  FLIGHT SAFETY/1(Safety Log) -> Safety log/1
  height signal/1 -> Display/1, FSM MONITOR/8(Height Signals (m) [4])
  Constant/1 -> FLIGHT SAFETY/3(Communication Loss)

== system Commander_Stabilizer_Qdrone_wTrajTEMP/motor command mapper ==
  Generalized commands : Inport
  arm : Inport  Port=2
  low battery : Inport  Port=3
  Constant : Constant
  Linear Thrust : control_library/Linear Thrust  SystemSampleTime=-1
  Maximum Command Authority : Saturate  UpperLimit=[1 1 1 1]  LowerLimit=[0 0 0 0]
  Motor command modulator : control_library/Motor command modulator  Commented=on  SystemSampleTime=-1
  Scope : Scope
  Set commands : Subsystem
  motor log : Outport
  wires:
  Maximum Command Authority/1 -> Set commands/1(Motor Cmd (%) [4]), motor log/1
  Generalized commands/1 -> Linear Thrust/1
  Constant/1 -> Linear Thrust/Enable
  arm/1 -> Set commands/2(Arm (0,1))
  low battery/1 -> Set commands/3(low battery)
  Linear Thrust/1 -> Scope/1, Maximum Command Authority/1

== system Commander_Stabilizer_Qdrone_wTrajTEMP/Communication1/Detect Communication Loss ==
  note: Stream Loss: Check if the state is 2 and error is positive (error codes are negative). Otherwise issue a communication error.
      | OR
      | Data Loss: Check if the data is stale for a while (this is required because a connected stream may publish no new data). If stale, issue a communication error.
  State : Inport
  Error : Inport  Port=2
  Data Out : Inport  Port=3
  Clock1 : Clock
  Communication Loss : Scope  NumInputPorts=2
  Data Type Conversion4 : DataTypeConversion
  Grab mission server time to detect flat lines : Selector  InputPortWidth=16  IndexOptions=Index vector (dialog)  Indices=[16]  OutputSizes=1
  Logical Operator4 : Logic  Operator=OR  AllPortsSameDT=off  OutDataTypeStr=boolean
  MATLAB Function : MATLAB Function  TreatAsAtomicUnit=on
  Terminator3 : Terminator
  Terminator5 : Terminator
  Threshold1 : quarc_library/Discontinuities/Threshold  operator=>=  param_src=Specify via dialog  threshold=0.5  duration=0.1
      settings: SourceProductName=QUARC Targets
  Threshold2 : quarc_library/Discontinuities/Threshold  operator=>=  param_src=Specify via dialog  threshold=0.5  duration=0.5
      settings: SourceProductName=QUARC Targets
  Communication Issue : Outport
  wires:
  Threshold2/1 -> Communication Loss/2, Logical Operator4/2
  Logical Operator4/1 -> Data Type Conversion4/1
  Threshold1/2 -> Terminator3/1
  MATLAB Function/2(data_loss) -> Threshold2/1
  MATLAB Function/1(stream_connection_loss) -> Threshold1/1
  Clock1/1 -> MATLAB Function/1(time)
  Threshold2/2 -> Terminator5/1
  Threshold1/1 -> Communication Loss/1, Logical Operator4/1
  Grab mission server time to detect flat lines/1 -> MATLAB Function/4(ms_time)
  Data Out/1 -> Grab mission server time to detect flat lines/1
  State/1 -> MATLAB Function/2(state)
  Error/1 -> MATLAB Function/3(error)
  Data Type Conversion4/1 -> Communication Issue/1

== system Commander_Stabilizer_Qdrone_wTrajTEMP/DAQ /Check Battery level ==
  Battery level : Inport
  Compare To Constant : simulink/Logic and Bit Operations/Compare To Constant  relop=<=  const=10.5  OutDataTypeStr=boolean
  Compare To Constant1 : simulink/Logic and Bit Operations/Compare To Constant  relop=>  const=0.5  OutDataTypeStr=boolean
  Data Type Conversion : DataTypeConversion
  Data Type Conversion1 : DataTypeConversion
  Logical Operator : Logic  AllPortsSameDT=off  OutDataTypeStr=boolean
  Terminator : Terminator
  Threshold : quarc_library/Discontinuities/Threshold  operator=>=  param_src=Specify via dialog  threshold=0.5  duration=0.1
      settings: SourceProductName=The database C:\Users\user\AppData\Roaming\MathWorks\MATLAB\R2017a\slblocks_master.db is locked, or a table in the database is locked. (database is locked)
  Low Battery : Outport
  wires:
  Threshold/2 -> Terminator/1
  Battery level/1 -> Compare To Constant1/1, Compare To Constant/1
  Threshold/1 -> Logical Operator/2
  Logical Operator/1 -> Data Type Conversion1/1
  Compare To Constant1/1 -> Logical Operator/1
  Compare To Constant/1 -> Data Type Conversion/1
  Data Type Conversion/1 -> Threshold/1
  Data Type Conversion1/1 -> Low Battery/1

== system Commander_Stabilizer_Qdrone_wTrajTEMP/DAQ /Sensor Failure Monitoring ==
  note: Check for no data condition (flat-line zero) from any of the onboard sensors
  Gyro Data [3] : Inport
  Accel Data [3]1 : Inport  Port=2
  Data Type Conversion1 : DataTypeConversion
  Data Type Conversion2 : DataTypeConversion
  Data Type Conversion4 : DataTypeConversion
  Logical Operator : Logic  Operator=OR  Inputs=1  AllPortsSameDT=off  OutDataTypeStr=boolean
  Mux : Mux  Inputs=2
  Sensor Failure (Accelerometer) : Subsystem
  Sensor Failure (Gyroscope) : Subsystem
  Sensor Failure : Outport
  wires:
  Accel Data [3]1/1 -> Sensor Failure (Accelerometer)/1(Sensor Input)
  Sensor Failure (Gyroscope)/1(Sensor Fault) -> Data Type Conversion2/1
  Sensor Failure (Accelerometer)/1(Sensor Fault) -> Data Type Conversion1/1
  Mux/1 -> Logical Operator/1
  Data Type Conversion2/1 -> Mux/1
  Data Type Conversion1/1 -> Mux/2
  Gyro Data [3]/1 -> Sensor Failure (Gyroscope)/1(Sensor Input)
  Logical Operator/1 -> Data Type Conversion4/1
  Data Type Conversion4/1 -> Sensor Failure/1

== system Commander_Stabilizer_Qdrone_wTrajTEMP/Estimation /Pose Rate Estimation ==
  note: Second order filter + Derivative
  note: Generate Pose Rate Approximation
  note: Improve Position Rate Estimate
  note: Complementary Filter implementation (similar to those in the Stabilizer module)
  note: The complementary filter uses an accurate but noisy pose rate approximation to correct the drifting integral of the fast accelerometer readings to yield an accurate and fast pose rate estimate.
  IF Vehicle Acceleration (m/s/s) [3] : Inport
  IF Pose Measurement (m) [3] : Inport  Port=2
  Reset : Inport  Port=3
  Integrator6 : Integrator
  Integrator7 : Integrator  ExternalReset=rising
  Ki3 : Gain  Gain=0.1
  Kp3 : Gain  Gain=4
  Second-Order Low-Pass Filter : quarc_library/Continuous/Second-Order Low-Pass Filter  params_source=External (input ports)  input_width=1  input_zeta=1  input_init=0
  Sum8 : Sum  Inputs=|-+
  Sum9 : Sum  Inputs=+--
  Terminator1 : Terminator
  wn : Constant  Value=50
  zt : Constant
  IF Pose Rate Estimate (m/s) [3] : Outport
  wires:
  Reset/1 -> Integrator7/2
  Integrator7/1 -> Sum9/3
  Kp3/1 -> Sum9/2
  Ki3/1 -> Integrator7/1
  Sum8/1 -> Kp3/1, Ki3/1
  Sum9/1 -> Integrator6/1
  Integrator6/1 -> Sum8/2, IF Pose Rate Estimate (m/s) [3]/1
  wn/1 -> Second-Order Low-Pass Filter/2
  Second-Order Low-Pass Filter/1 -> Terminator1/1
  Second-Order Low-Pass Filter/2 -> Sum8/1
  zt/1 -> Second-Order Low-Pass Filter/3
  IF Vehicle Acceleration (m/s/s) [3]/1 -> Sum9/1
  IF Pose Measurement (m) [3]/1 -> Second-Order Low-Pass Filter/4, Second-Order Low-Pass Filter/1

== system Commander_Stabilizer_Qdrone_wTrajTEMP/Estimation /Transform from Body Frame to Inertial Frame ==
  note: Accelerometer Reading + Gravity = Vehicle Acceleration
  BF Net Acceleration (m/s/s) [3] : Inport
  IF_R_BF : Inport  Port=2
  Display : Display
  Product : Product  Multiplication=Matrix(*)
  gravity correction : Bias  Bias=[0 0 -9.81]
  HF Vehicle Acceleration (m/s/s) [3] : Outport
  wires:
  gravity correction/1 -> Display/1, HF Vehicle Acceleration (m/s/s) [3]/1  "IF Vehicle Acceleration"
  IF_R_BF/1 -> Product/1
  BF Net Acceleration (m/s/s) [3]/1 -> Product/2
  Product/1 -> gravity correction/1  "IF Accelerometer Reading"

== system Commander_Stabilizer_Qdrone_wTrajTEMP/Estimation /Transform from Inertial Frame to Horizon Frame ==
  HF_R_IF : Inport
  IF Pose Measurement (m) [3] : Inport  Port=2
  IF Pose Command (m) [3] : Inport  Port=3
  IF pose rate command (m/s) [3] : Inport  Port=4
  IF Desired Acc : Inport  Port=5
  Product{1..4} (4 alike) : Product  Multiplication=Matrix(*)
  HF Pose Estimate (m) [3] : Outport
  HF Pose Command (m) [3] : Outport  Port=2
  HF Pose Rate command (m/s) [3] : Outport  Port=3
  tag scope: acc_cmd_8sh_HF=global
  wires:
  IF Pose Command (m) [3]/1 -> Product1/2
  Product2/1 -> HF Pose Estimate (m) [3]/1  "HF Position Measurement"
  Product1/1 -> HF Pose Command (m) [3]/1  "HF Position Command"
  HF_R_IF/1 -> Product4/1, Product3/1, Product2/1, Product1/1
  IF pose rate command (m/s) [3]/1 -> Product3/2
  Product3/1 -> HF Pose Rate command (m/s) [3]/1  "HF Position Measurement"
  IF Pose Measurement (m) [3]/1 -> Product2/2
  IF Desired Acc/1 -> Product4/2
  Product4/1 -> [acc_cmd_8sh_HF]  "HF Desired Acc"

== system Commander_Stabilizer_Qdrone_wTrajTEMP/Estimation /acc_calibration ==
  In1 : Inport
  Constant : Constant  Value=acc_calib.offsets
  Constant1 : Constant  Value=inv(acc_calib.gains)
  Constant2 : Constant  Value=acc_calib.R_a2b
  Matrix Multiply : Product  Multiplication=Matrix(*)
  Matrix Multiply1 : Product  Multiplication=Matrix(*)
  Sum : Sum  Inputs=|+-
  Out1 : Outport
  wires:
  In1/1 -> Sum/1
  Sum/1 -> Matrix Multiply/2
  Constant/1 -> Sum/2
  Constant1/1 -> Matrix Multiply/1
  Matrix Multiply/1 -> Matrix Multiply1/2
  Matrix Multiply1/1 -> Out1/1
  Constant2/1 -> Matrix Multiply1/1

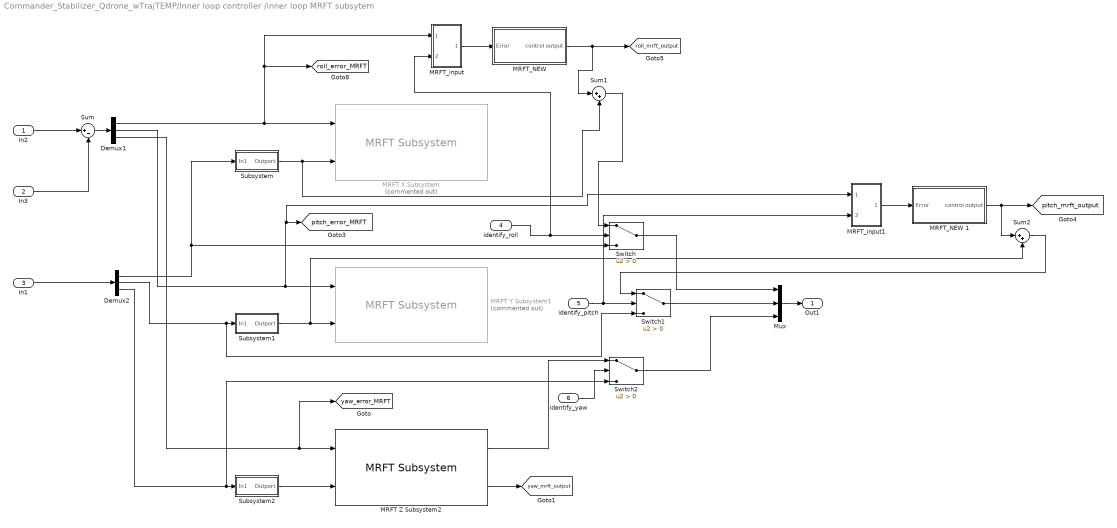
== system Commander_Stabilizer_Qdrone_wTrajTEMP/Inner loop controller /inner loop MRFT subsytem ==
  In2 : Inport
  In3 : Inport  Port=2
  In1 : Inport  Port=3
  identify_roll : Inport  Port=4
  "identify_pitch " : Inport  Port=5
  identify_yaw : Inport  Port=6
  Demux1 : Demux  Outputs=3
  Demux2 : Demux  Outputs=3
  MRFT X Subsystem : control_library/MRFT Subsystem  Commented=on  h_relay=0.3  beta=-0.73
  MRFT Y Subsystem1 : control_library/MRFT Subsystem  Commented=on  h_relay=0.3  beta=-0.737
  MRFT Z Subsystem2 : control_library/MRFT Subsystem  h_relay=0.3  beta=0.5
  "MRFT_NEW " : Subsystem
  MRFT_NEW 1 : Subsystem
  MRFT_input : Subsystem
  MRFT_input1 : Subsystem
  Mux : Mux  Inputs=3
  Subsystem : Subsystem
  Subsystem1 : Subsystem
  Subsystem2 : Subsystem
  Sum : Sum  Inputs=|+-
  Sum1 : Sum  Inputs=|++
  Sum2 : Sum  Inputs=|++
  Switch : Switch  Criteria=u2 > Threshold
  Switch1 : Switch  Criteria=u2 > Threshold
  Switch2 : Switch  Criteria=u2 > Threshold
  Out1 : Outport
  tag scope: pitch_error_MRFT=global, pitch_mrft_output=global, roll_error_MRFT=global, roll_mrft_output=global, yaw_error_MRFT=global, yaw_mrft_output=global
  wires:
  In1/1 -> Demux2/1
  In2/1 -> Sum/1
  In3/1 -> Sum/2
  Sum/1 -> Demux1/1
  Demux1/1 -> MRFT_input/1(data), [roll_error_MRFT], MRFT X Subsystem/1
  Demux2/1 -> Subsystem/1(In1), Switch/3
  identify_roll/1 -> MRFT_input/2(switch), Switch/2
  Mux/1 -> Out1/1
  Switch/1 -> Mux/1
  Subsystem/1(Outport) -> Sum1/2, MRFT X Subsystem/2
  MRFT Z Subsystem2/1 -> Switch2/1
  Subsystem1/1(Outport) -> Sum2/2, MRFT Y Subsystem1/2
  Demux2/2 -> Switch1/3, Subsystem1/1(In1)
  Demux2/3 -> Switch2/3, Subsystem2/1(In1)
  Demux1/2 -> MRFT Y Subsystem1/1, MRFT_input1/1(data), [pitch_error_MRFT]
  Demux1/3 -> [yaw_error_MRFT], MRFT Z Subsystem2/1
  Subsystem2/1(Outport) -> MRFT Z Subsystem2/2
  Switch1/1 -> Mux/2
  Switch2/1 -> Mux/3
  "identify_pitch "/1 -> MRFT_input1/2(switch), Switch1/2
  identify_yaw/1 -> Switch2/2
  MRFT Z Subsystem2/2 -> [yaw_mrft_output]
  MRFT_input/1(Out1) -> "MRFT_NEW "/1(Error)
  "MRFT_NEW "/1(control output) -> Sum1/1, [roll_mrft_output]
  Sum1/1 -> Switch/1
  MRFT_input1/1(Out1) -> MRFT_NEW 1/1(Error)
  MRFT_NEW 1/1(control output) -> Sum2/1, [pitch_mrft_output]
  Sum2/1 -> Switch1/1

== system Commander_Stabilizer_Qdrone_wTrajTEMP/Outer loop/Subsystem ==
  Error : Inport
  Flag : Inport  Port=2
  Gain : Gain  Gain=5
  Integrator : Integrator  ExternalReset=either
  Memory : Memory
  Switch : Switch  Criteria=u2 > Threshold
  Bias : Outport
  wires:
  Error/1 -> Integrator/1
  Integrator/1 -> Gain/1
  Flag/1 -> Switch/2, Integrator/2
  Switch/1 -> Bias/1, [bias]
  [bias] -> Memory/1
  Gain/1 -> Switch/3
  Memory/1 -> Switch/1

== system Commander_Stabilizer_Qdrone_wTrajTEMP/Outer loop/Subsystem1 ==
  Error : Inport
  Flag : Inport  Port=2
  Gain : Gain  Gain=10
  Integrator : Integrator  ExternalReset=either
  Memory : Memory
  Switch : Switch  Criteria=u2 > Threshold
  Bias : Outport
  wires:
  [bias] -> Memory/1
  Switch/1 -> [bias], Bias/1
  Flag/1 -> Integrator/2, Switch/2
  Integrator/1 -> Gain/1
  Error/1 -> Integrator/1
  Gain/1 -> Switch/3
  Memory/1 -> Switch/1
